simulink library "golayLib"  (R2017a)
settings: Solver=ode45  StartTime=0.0  StopTime=10.0  RelTol=1e-3  EnableMultiTasking=on
values from neighbouring files (symbols this model uses):
  mult_pipeline = 1    [rev0BB_setup.m]
undefined symbols (not defined in the file): D_128, W_128
settings Model: Creator=cyarp  LastModifiedBy=cyarp
settings DataIOCC: LimitDataPoints=on  SaveFormat=Array
settings OptimizationCC: LifeSpan=inf
settings DebuggingCC: SolverPrmCheckMsg=warning  SFUnexpectedBacktrackingDiag=warning  SFNoUnconditionalDefaultTransitionDiag=warning  SFExecutionAtInitializationDiag=none
settings HardwareCC: ProdBitPerPointer=32  ProdBitPerSizeT=32  ProdBitPerPtrDiffT=32  ProdLargestAtomicFloat=None  ProdIntDivRoundTo=Undefined  ProdEndianess=Unspecified  ProdWordSize=32  ProdHWDeviceType=32-bit Generic
settings ModelReferenceCC: PropagateSignalLabelsOutOfModel=off
settings GRTTargetCC: TargetLangStandard=C89/C90 (ANSI)  GeneratePreprocessorConditionals=Disable all
settings ConfigComp: CovMetricSettings=dw  CovHtmlReporting=on  CovSaveCumulativeToWorkspaceVar=on  CovSaveSingleToWorkspaceVar=on  CovExternalEMLEnable=off  CovSFcnEnable=off

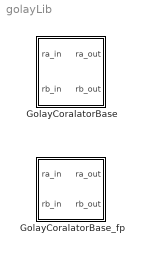
== system golayLib ==
  GolayCoralatorBase : Subsystem  mask(Golay Correlator Base){dSub=D_128(1), wSub=W_128(1)}
      mask prompts: dSub "D Parameter"; wSub "W Parameter"
      mask help: Base Unit of a Golay Correlator
  GolayCoralatorBase_fp : Subsystem  mask{dSub=0, wSub=0, mult=0}
      mask prompts: dSub "D Parameter"; wSub "W Parameter"; mult "Multiply Pipeline Delay"

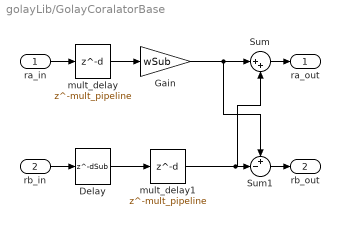
== system golayLib/GolayCoralatorBase ==
  ra_in : Inport  OutDataTypeStr=int16
  rb_in : Inport  Port=2  OutDataTypeStr=int16
  Delay : Delay  DelayLength=dSub  DelayLengthUpperLimit=1000  InitialCondition=0  DiagnosticForDelayLength=Error  UseCircularBuffer=on
  Gain : Gain  Gain=wSub  OutDataTypeStr=Inherit: Same as input
  Sum : Sum  Inputs=|++
  Sum1 : Sum  Inputs=+-|
  mult_delay : Delay  DelayLength=mult_pipeline
  mult_delay1 : Delay  DelayLength=mult_pipeline
  ra_out : Outport  OutDataTypeStr=int16
  rb_out : Outport  Port=2  OutDataTypeStr=int16
  wires:
  Sum/1 -> ra_out/1
  Sum1/1 -> rb_out/1
  rb_in/1 -> Delay/1
  Delay/1 -> mult_delay1/1
  Gain/1 -> Sum1/1, Sum/1
  mult_delay1/1 -> Sum/2, Sum1/2
  ra_in/1 -> mult_delay/1
  mult_delay/1 -> Gain/1

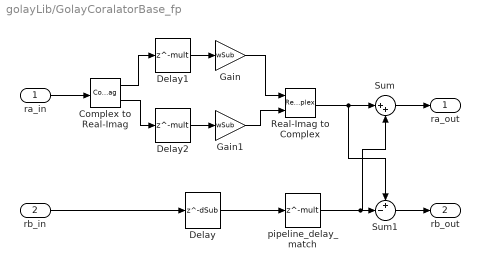
== system golayLib/GolayCoralatorBase_fp ==
  ra_in : Inport
  rb_in : Inport  Port=2
  Complex to Real-Imag : ComplexToRealImag
  Delay : Delay  DelayLength=dSub  DelayLengthUpperLimit=1000  InitialCondition=0  DiagnosticForDelayLength=Error  UseCircularBuffer=on
  Delay1 : Delay  DelayLength=mult  InitialCondition=0
  Delay2 : Delay  DelayLength=mult  InitialCondition=0
  Gain : Gain  Gain=wSub  OutDataTypeStr=Inherit: Same as input  ParamDataTypeStr=Inherit: Same as input
  Gain1 : Gain  Gain=wSub  OutDataTypeStr=Inherit: Same as input  ParamDataTypeStr=Inherit: Same as input
  Real-Imag to Complex : RealImagToComplex
  Sum : Sum  Inputs=|++
  Sum1 : Sum  Inputs=+-|
  pipeline_delay_match : Delay  DelayLength=mult
  ra_out : Outport
  rb_out : Outport  Port=2
  wires:
  Delay/1 -> pipeline_delay_match/1
  rb_in/1 -> Delay/1
  pipeline_delay_match/1 -> Sum/2, Sum1/2
  Real-Imag to Complex/1 -> Sum1/1, Sum/1
  ra_in/1 -> Complex to Real-Imag/1
  Sum1/1 -> rb_out/1
  Sum/1 -> ra_out/1
  Delay1/1 -> Gain/1
  Gain/1 -> Real-Imag to Complex/1
  Complex to Real-Imag/1 -> Delay1/1
  Delay2/1 -> Gain1/1
  Gain1/1 -> Real-Imag to Complex/2
  Complex to Real-Imag/2 -> Delay2/1
